simulink model "Doblependulo"  (R2024a)
settings: Solver=VariableStepAuto  StartTime=0.0  StopTime=10.0  RelTol=1e-3
values from neighbouring files (symbols this model uses):
  g = 9.81    [exp1.m]
  l1 = 0.3    [exp1.m]
  l2 = 0.25    [exp1.m]
  m1 = 0.2    [exp1.m]
  m2 = 0.1    [exp1.m]
settings Model: Creator=Braulio Ramíreza  LastModifiedBy=Braulio Ramíreza

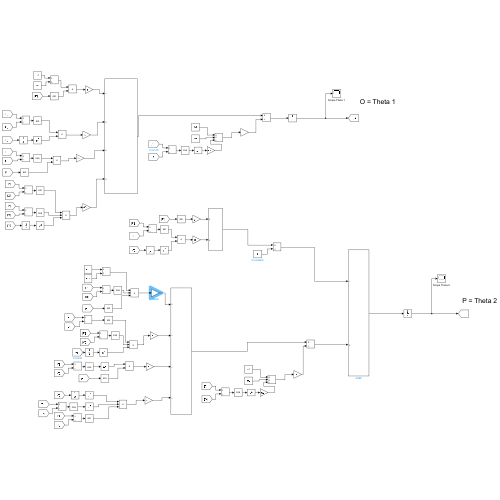
[thumbnail: Simulink's stored preview of the top-level diagram]
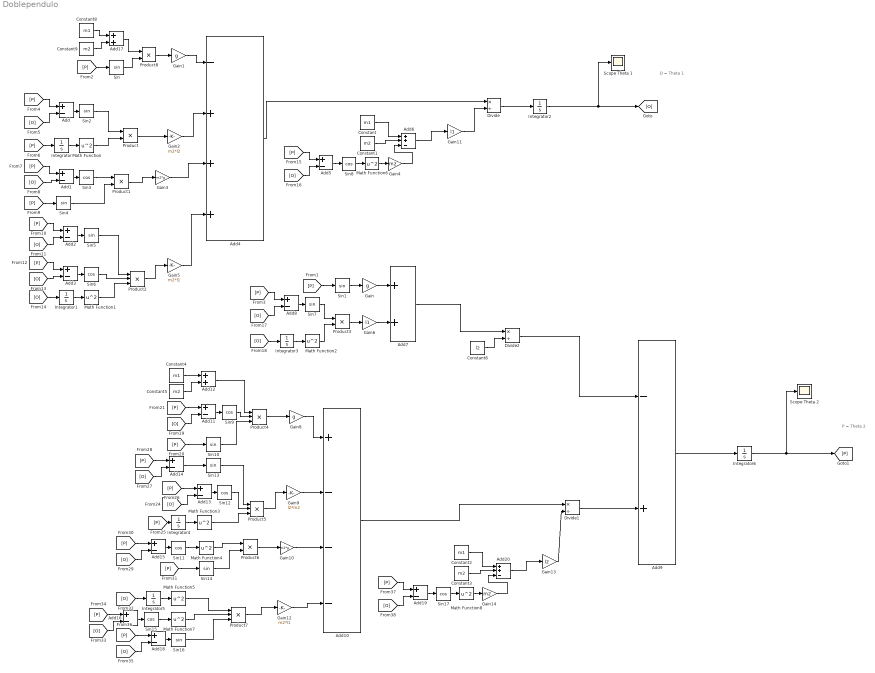
== system Doblependulo ==
  note: P = Theta 2
  note: O = Theta 1
  Add{,1..3,5,8,11,13..16,18..19} (13 alike) : Sum  Inputs=+-
  Add10 : Sum  Inputs=+---
  Add12 : Sum
  Add17 : Sum
  Add20 : Sum  Inputs=++-
  Add4 : Sum  Inputs=-+++
  Add6 : Sum  Inputs=++-
  Add7 : Sum
  Add9 : Sum  Inputs=-+
  Constant{,2,4,8} (4 alike) : Constant  Value=m1
  Constant{1,3,5,9} (4 alike) : Constant  Value=m2
  Constant6 : Constant  Value=l2
  Divide : Product  Inputs=*/
  Divide1 : Product  Inputs=*/
  Divide2 : Product  Inputs=*/
  Gain : Gain  Gain=g
  Gain1 : Gain  Gain=g
  Gain10 : Gain  Gain=m2*g
  Gain11 : Gain  Gain=l1
  Gain12 : Gain  Gain=m2*l1
  Gain13 : Gain  Gain=l2
  Gain14 : Gain  Gain=m2
  Gain2 : Gain  Gain=m2*l2
  Gain3 : Gain  Gain=m2*g
  Gain4 : Gain  Gain=m2
  Gain5 : Gain  Gain=m2*l1
  Gain6 : Gain  Gain=l1
  Gain8 : Gain  Gain=g
  Gain9 : Gain  Gain=l2*m2
  Integrator{,1..5} (6 alike) : Integrator
  Integrator6 : Integrator  InitialCondition=(35*pi)/180
  Math Function{,1..8} (9 alike) : Math  Operator=square
  Product{,1,3,6,8} (5 alike) : Product
  Product{2,4..5,7} (4 alike) : Product  Inputs=3
  Scope Theta 1 : Scope
  Scope Theta 2 : Scope
  Sin{,1..2,4..5,7,10,13..14,16} (10 alike) : Trigonometry
  Sin{3,6,8..9,11..12,15,17} (8 alike) : Trigonometry  Operator=cos
  wires:
  [P] -> Sin/1
  Sin/1 -> Product8/2
  [P] -> Add/1
  [O] -> Add/2
  Add/1 -> Sin2/1
  [P] -> Integrator/1
  Integrator/1 -> Math Function/1
  Math Function/1 -> Product/2
  Sin2/1 -> Product/1
  Gain2/1 -> Add4/2
  Product/1 -> Gain2/1
  [O] -> Add1/2
  [P] -> Add1/1
  Add1/1 -> Sin3/1
  Sin3/1 -> Product1/1
  [P] -> Sin4/1
  Sin4/1 -> Product1/2
  Product1/1 -> Gain3/1
  Gain3/1 -> Add4/3
  [O] -> Add2/2
  [P] -> Add2/1
  Add2/1 -> Sin5/1
  Add3/1 -> Sin6/1
  [P] -> Add3/1
  [O] -> Add3/2
  Integrator1/1 -> Math Function1/1
  [O] -> Integrator1/1
  Math Function1/1 -> Product2/3
  Sin6/1 -> Product2/2
  Sin5/1 -> Product2/1
  [P] -> Add5/1
  [O] -> Add5/2
  Add5/1 -> Sin8/1
  Add4/1 -> Divide/1
  Constant1/1 -> Add6/2
  Constant/1 -> Add6/1
  Gain4/1 -> Add6/3
  Divide/1 -> Integrator2/1
  Product2/1 -> Gain5/1
  Gain5/1 -> Add4/4
  Add6/1 -> Gain11/1
  Gain11/1 -> Divide/2
  Sin8/1 -> Math Function6/1
  Math Function6/1 -> Gain4/1
  Constant8/1 -> Add17/1
  Constant9/1 -> Add17/2
  Add17/1 -> Product8/1
  Product8/1 -> Gain1/1
  Gain1/1 -> Add4/1
  [P] -> Sin1/1
  Sin1/1 -> Gain/1
  Gain/1 -> Add7/1
  [P] -> Add8/1
  [O] -> Add8/2
  Add8/1 -> Sin7/1
  [O] -> Integrator3/1
  Integrator3/1 -> Math Function2/1
  Sin7/1 -> Product3/1
  Math Function2/1 -> Product3/2
  Product3/1 -> Gain6/1
  Gain6/1 -> Add7/2
  Add7/1 -> Divide2/1
  Sin10/1 -> Product4/3
  Add11/1 -> Sin9/1
  [P] -> Sin10/1
  [O] -> Add11/2
  [P] -> Add11/1
  Sin9/1 -> Product4/2
  Product4/1 -> Gain8/1
  Gain8/1 -> Add10/1
  Constant4/1 -> Add12/1
  Constant5/1 -> Add12/2
  Add12/1 -> Product4/1
  Add13/1 -> Sin12/1
  [P] -> Add13/1
  [O] -> Add13/2
  [O] -> Add14/2
  Sin12/1 -> Product5/2
  [P] -> Integrator4/1
  [P] -> Add14/1
  Add14/1 -> Sin13/1
  Sin13/1 -> Product5/1
  Integrator4/1 -> Math Function3/1
  Math Function3/1 -> Product5/3
  Product5/1 -> Gain9/1
  Gain9/1 -> Add10/2
  [O] -> Add15/2
  [P] -> Add15/1
  Add15/1 -> Sin11/1
  Sin11/1 -> Math Function4/1
  [P] -> Sin14/1
  Sin14/1 -> Product6/2
  Math Function4/1 -> Product6/1
  Integrator5/1 -> Math Function5/1
  [O] -> Integrator5/1
  Add18/1 -> Sin16/1
  Sin15/1 -> Math Function7/1
  [O] -> Add16/2
  Add16/1 -> Sin15/1
  Sin16/1 -> Product7/3
  Math Function7/1 -> Product7/2
  [P] -> Add16/1
  [O] -> Add18/2
  [P] -> Add18/1
  Math Function5/1 -> Product7/1
  Product6/1 -> Gain10/1
  Gain10/1 -> Add10/3
  Product7/1 -> Gain12/1
  Gain12/1 -> Add10/4
  [P] -> Add19/1
  Gain13/1 -> Divide1/2
  Add19/1 -> Sin17/1
  Add20/1 -> Gain13/1
  [O] -> Add19/2
  Sin17/1 -> Math Function8/1
  Constant3/1 -> Add20/2
  Math Function8/1 -> Gain14/1
  Constant2/1 -> Add20/1
  Gain14/1 -> Add20/3
  Add10/1 -> Divide1/1
  Divide1/1 -> Add9/2
  Add9/1 -> Integrator6/1
  Constant6/1 -> Divide2/2
  Divide2/1 -> Add9/1
  Integrator2/1 -> Scope Theta 1/1, [O]
  Integrator6/1 -> Scope Theta 2/1, [P]
